simulink model "sedemo_async_stateflow"  (Simulink 7.5)
settings: Solver=VariableStepDiscrete  StartTime=0.0  StopTime=30  MaxStep=inf  RelTol=1e-3
libraries: simulink x3, simeventstranslate1 x3, simeventsinfo x1
settings Model: Creator=The MathWorks Inc.
settings DataIOCC: SaveOutput=off  SaveTime=off
settings OptimizationCC: InitFltsAndDblsToZero=on  EfficientMapNaN2IntZero=off
settings DebuggingCC: AlgebraicLoopMsg=error  SaveWithParameterizedLinksMsg=none  SignalResolutionControl=TryResolveAllWithWarning  SolverPrmCheckMsg=none  StrictBusMsg=Warning
settings GRTTargetCC: TargetFcnLib=ansi_tfl_tmw.mat
settings SimEventsCC: propDiagAttribOutput=1  propDiagFcnCallOutput=1  propDiagStatOutput=0

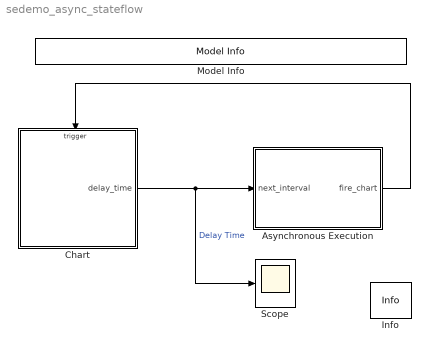
== system sedemo_async_stateflow ==
  Asynchronous Execution : Subsystem
  Chart : Stateflow chart  TreatAsAtomicUnit=on
      settings: PropExecContextOutsideSubsystem=on
  Info : simeventsinfo/Info  SystemSampleTime=-1
  Model Info : simulink/Model-Wide Utilities/Model Info  SystemSampleTime=-1  InitialBlockCM=None  BlockCM=None  Frame=off  DisplayStringWithTags=Asynchronous Execution of a Stateflow Chart  HorizontalTextAlignment=Center  LeftAlignmentValue=0.5  SourceBlockDiagram=sedemo_async_stateflow  TagMaxNumber=20
  Scope : Scope
      settings: TickLabels=on  TimeRange=30  YMin=0  YMax=10
  wires:
  Asynchronous Execution/1(fire_chart) -> Chart/Trigger
  Chart/1(delay_time) -> Asynchronous Execution/1(next_interval), Scope/1  "Delay Time"

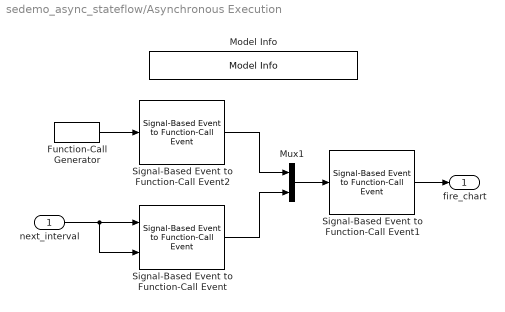
== system sedemo_async_stateflow/Asynchronous Execution ==
  next_interval : Inport
  Function-Call Generator : simulink/Ports & Subsystems/Function-Call Generator  sample_time=1e100  numberOfIterations=1
  Model Info : simulink/Model-Wide Utilities/Model Info  SystemSampleTime=-1  InitialBlockCM=None  BlockCM=None  Frame=off  DisplayStringWithTags=Delayed Function Calls  HorizontalTextAlignment=Center  LeftAlignmentValue=0.5  SourceBlockDiagram=sedemo_delayed_stateflow  TagMaxNumber=20
  Mux1 : Mux  Inputs=2
  Signal-Based Event to Function-Call Event : simeventstranslate1/Signal-Based Event to Function-Call Event  Priority=1  SystemSampleTime=-1  GenerateFunctionCallUpon=Sample time hit from port ts  SignalEdgeOption=Either  EnableE1Port=off  EnableF2Port=off  EnableE2Port=off  SpecifyEventPriority=on  PriorityFunctionCall=200  FunctionCallDelayFrom=Signal port t  DelayFunctionCall=0  StatNumberF1Calls=Off  StatNumberF2Calls=Off  MaskBlockType=none
  Signal-Based Event to Function-Call Event1 : simeventstranslate1/Signal-Based Event to Function-Call Event  Priority=1  SystemSampleTime=-1  GenerateFunctionCallUpon=Function call from port fcn  SignalEdgeOption=Either  EnableE1Port=off  EnableF2Port=off  EnableE2Port=off  SpecifyEventPriority=off  PriorityFunctionCall=200  FunctionCallDelayFrom=Signal port t  DelayFunctionCall=0  StatNumberF1Calls=Off  StatNumberF2Calls=Off  MaskBlockType=none
  Signal-Based Event to Function-Call Event2 : simeventstranslate1/Signal-Based Event to Function-Call Event  Priority=1  SystemSampleTime=-1  GenerateFunctionCallUpon=Function call from port fcn  SignalEdgeOption=Either  EnableE1Port=off  EnableF2Port=off  EnableE2Port=off  SpecifyEventPriority=off  PriorityFunctionCall=200  FunctionCallDelayFrom=Signal port t  DelayFunctionCall=0  StatNumberF1Calls=Off  StatNumberF2Calls=Off  MaskBlockType=none
  fire_chart : Outport
  wires:
  Function-Call Generator/1 -> Signal-Based Event to Function-Call Event2/1
  Signal-Based Event to Function-Call Event1/1 -> fire_chart/1
  next_interval/1 -> Signal-Based Event to Function-Call Event/1, Signal-Based Event to Function-Call Event/2
  Signal-Based Event to Function-Call Event2/1 -> Mux1/1
  Signal-Based Event to Function-Call Event/1 -> Mux1/2
  Mux1/1 -> Signal-Based Event to Function-Call Event1/1

== stateflow chart Chart ==
  settings: sampleTime=1
  state Active
    entry:delay_time = delay_time + 1;
  state End
  note: Stateflow Chart Logic
  Active -> End [order 1] : [delay_time > 5]
  (default) -> Active : {delay_time=0;}
  Active -> Active [order 2] : event_in
  data: delay_time output double
  events: event_in input FUNCTION_CALL_EVENT
